simulink model "triggered"  (R2024a)
settings: Solver=FixedStepDiscrete  StartTime=0.0  StopTime=10.0  FixedStep=0.5  RelTol=1e-3
settings Model: Creator=DELL  LastModifiedBy=DELL
settings OptimizationCC: DefaultParameterBehavior=Inlined  EnhancedBackFolding=on  PassReuseOutputArgsAs=Individual arguments  ZeroExternalMemoryAtStartup=off  ZeroInternalMemoryAtStartup=off  OptimizeBlockOrder=speed  DifferentSizesBufferReuse=on  OptimizationCustomize=off  EfficientTunableParamExpr=on
settings DebuggingCC: ParameterTunabilityLossMsg=error
settings SFSimCC: MATLABDynamicMemAlloc=off
settings RTWCC: Description=Embedded Coder  SystemTargetFile=ert.tlc  TemplateMakefile=ert_default_tmf
settings CodeAppCC: ForceParamTrailComments=on  IgnoreCustomStorageClasses=off  OperatorAnnotations=on  SimulinkDataObjDesc=on  SFDataObjDesc=on  InsertBlockDesc=on
settings ERTTargetCC: TargetLangStandard=C99 (ISO)  GenerateSampleERTMain=on  InlinedParameterPlacement=NonHierarchical  ERTCustomFileTemplate=example_file_process.tlc

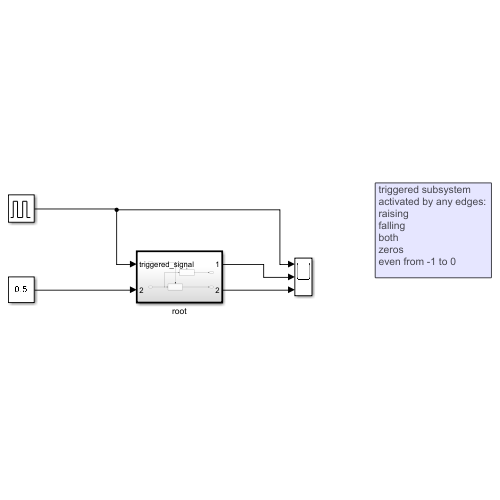
[thumbnail: Simulink's stored preview of the top-level diagram]
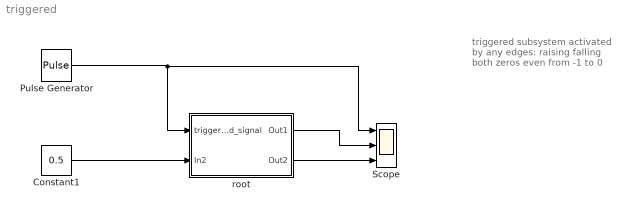
== system triggered ==
  note: triggered subsystem
      | activated by any edges:
      | raising
      | falling
      | both
      | zeros
      | even from -1 to 0
  Constant1 : Constant  Value=0.5
  Pulse Generator : DiscretePulseGenerator  PulseType=Time based  Period=1  PulseWidth=50
  Scope : Scope  NumInputPorts=3
  root : Subsystem  TreatAsAtomicUnit=on
      settings: RTWSystemCode=Nonreusable function  RTWFcnNameOpts=Use subsystem name
  wires:
  Pulse Generator/1 -> Scope/1, root/1(triggered_signal)
  Constant1/1 -> root/2(In2)
  root/1(Out1) -> Scope/2
  root/2(Out2) -> Scope/3

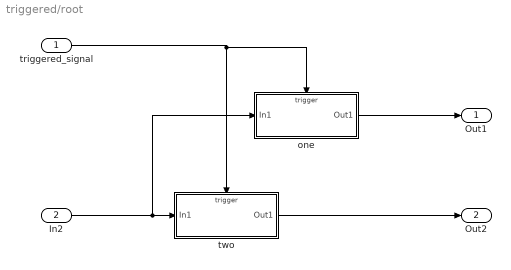
== system triggered/root ==
  triggered_signal : Inport
  In2 : Inport  Port=2
  one : Subsystem  TreatAsAtomicUnit=on
      settings: RTWSystemCode=Nonreusable function
  two : Subsystem  TreatAsAtomicUnit=on
      settings: RTWSystemCode=Nonreusable function
  Out1 : Outport
  Out2 : Outport  Port=2
  wires:
  In2/1 -> one/1(In1), two/1(In1)
  one/1(Out1) -> Out1/1
  triggered_signal/1 -> two/Trigger, one/Trigger
  two/1(Out1) -> Out2/1

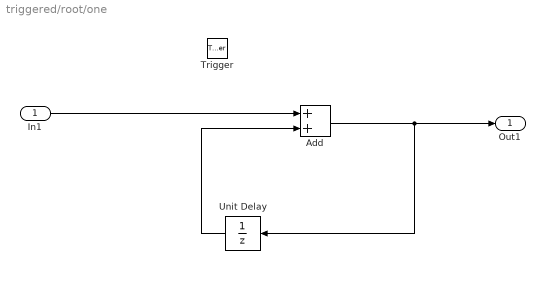
== system triggered/root/one ==
  In1 : Inport
  Trigger : TriggerPort  VariantControl=(inherit)  PortDimensions=1
  Add : Sum
  Unit Delay : UnitDelay  SampleTime=-1  HasFrameUpgradeWarning=on
  Out1 : Outport
  wires:
  In1/1 -> Add/1
  Unit Delay/1 -> Add/2
  Add/1 -> Unit Delay/1, Out1/1

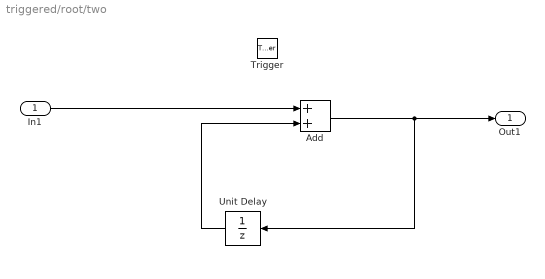
== system triggered/root/two ==
  In1 : Inport
  Trigger : TriggerPort  TriggerType=falling  VariantControl=(inherit)  PortDimensions=1
  Add : Sum
  Unit Delay : UnitDelay  SampleTime=-1  HasFrameUpgradeWarning=on
  Out1 : Outport
  wires:
  Add/1 -> Out1/1, Unit Delay/1
  Unit Delay/1 -> Add/2
  In1/1 -> Add/1
